simulink model "Example_2_Open"  (Simulink 8.3)
settings: Solver=ode45  StartTime=0.0  StopTime=50  RelTol=1e-3
libraries: simulink x1
settings Model: Creator=NeuControl  LastModifiedBy=Li Jinghao
settings DataIOCC: SignalLoggingSaveFormat=Dataset
settings DebuggingCC: UnderspecifiedInitializationDetection=Simplified  StateNameClashWarn=none
settings GRTTargetCC: CombineOutputUpdateFcns=on  GRTInterface=off

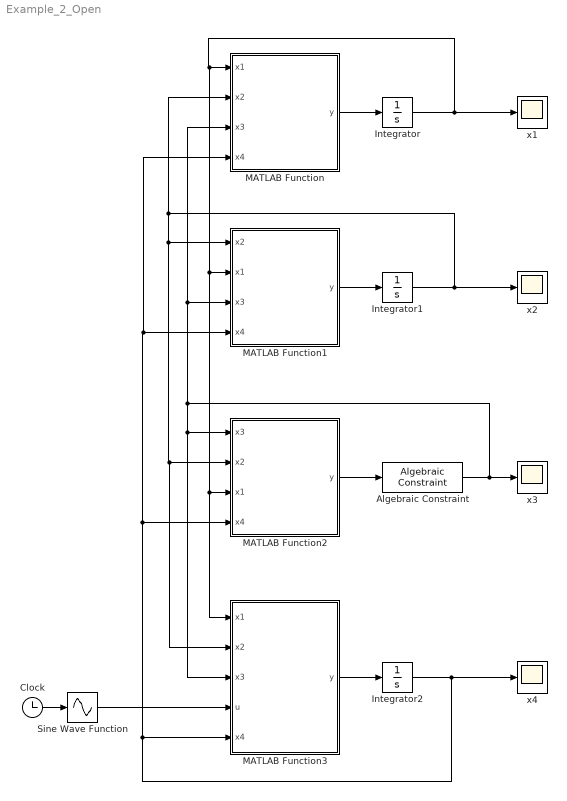
== system Example_2_Open ==
  Algebraic Constraint : simulink/Math Operations/Algebraic Constraint  z0=0
  Clock : Clock
  Integrator : Integrator  InitialCondition=0.5
  Integrator1 : Integrator  InitialCondition=-1
  Integrator2 : Integrator  InitialCondition=2
  MATLAB Function : MATLAB Function  TreatAsAtomicUnit=on
  MATLAB Function1 : MATLAB Function  TreatAsAtomicUnit=on
  MATLAB Function2 : MATLAB Function  TreatAsAtomicUnit=on
  MATLAB Function3 : MATLAB Function  TreatAsAtomicUnit=on
  Sine Wave Function : Sin  TimeSource=Use external signal  Phase=pi/2  SampleTime=0
  x{1..4} (4 alike) : Scope
      x1 settings: SaveName=x1
      x2 settings: SaveName=x2
      x3 settings: SaveName=x3
      x4 settings: SaveName=x4
  wires:
  Integrator/1 -> MATLAB Function3/1(x1), MATLAB Function2/3(x1), MATLAB Function1/2(x1), MATLAB Function/1(x1), x1/1
  MATLAB Function/1(y) -> Integrator/1
  Integrator1/1 -> MATLAB Function/2(x2), MATLAB Function1/1(x2), MATLAB Function3/2(x2), MATLAB Function2/2(x2), x2/1
  MATLAB Function1/1(y) -> Integrator1/1
  Algebraic Constraint/1 -> x3/1, MATLAB Function/3(x3), MATLAB Function1/3(x3), MATLAB Function3/3(x3), MATLAB Function2/1(x3)
  MATLAB Function2/1(y) -> Algebraic Constraint/1
  Integrator2/1 -> x4/1, MATLAB Function3/5(x4), MATLAB Function/4(x4), MATLAB Function1/4(x4), MATLAB Function2/4(x4)
  MATLAB Function3/1(y) -> Integrator2/1
  Clock/1 -> Sine Wave Function/1
  Sine Wave Function/1 -> MATLAB Function3/4(u)

== matlab function MATLAB Function1 ==
  data: x2 input double; x1 input double; y output double; x3 input double; x4 input double
function y = fcn(x2,x1,x3,x4)
%#codegen

gamma=1;
w1=exp(-0.5*(0.5*(x1+5))^2);
w2=exp(-0.5*(0.5*x1)^2);
w3=exp(-0.5*(0.5*(x1-5))^2);
v1=w1/(w1+w2+w3);
v2=w2/(w1+w2+w3);
v3=1-v1-v2;
A1=[-0.5 -0.5 -1 1];
A2=[0.5 -1 0 0.5];
A3=[gamma -1 1 0];
A=v1*A1+v2*A2+v3*A3;
x=[x1;x2;x3;x4];
y = A*x;

== matlab function MATLAB Function ==
  data: x1 input double; y output double; x2 input double; x3 input double; x4 input double
function y = fcn(x1,x2,x3,x4)
%#codegen

beta=-2;
gamma=1;
w1=exp(-0.5*(0.5*(x1+5))^2);
w2=exp(-0.5*(0.5*x1)^2);
w3=exp(-0.5*(0.5*(x1-5))^2);
v1=w1/(w1+w2+w3);
v2=w2/(w1+w2+w3);
v3=1-v1-v2;
A1=[-1 beta 1 -0.5];
A2=[gamma 0.5 0 1];
A3=[-1 beta 0 1];
A=v1*A1+v2*A2+v3*A3;
x=[x1;x2;x3;x4];
y = A*x;

== matlab function MATLAB Function2 ==
  data: x3 input double; x2 input double; x1 input double; y output double; x4 input double
function y = fcn(x3,x2,x1,x4)
%#codegen

w1=exp(-0.5*(0.5*(x1+5))^2);
w2=exp(-0.5*(0.5*x1)^2);
w3=exp(-0.5*(0.5*(x1-5))^2);
v1=w1/(w1+w2+w3);
v2=w2/(w1+w2+w3);
v3=1-v1-v2;
A1=[0 0 -1 1];
A2=[1 0 -1 0.5];
A3=[0 1 -1 1];
A=v1*A1+v2*A2+v3*A3;
x=[x1;x2;x3;x4];
y = A*x;

== matlab function MATLAB Function3 ==
  data: x1 input double; x2 input double; x3 input double; u input double; x4 input double; y output double
function y = fcn(x1,x2,x3,u,x4)
%#codegen


A=[0.5 1 -1.5 1];
x=[x1;x2;x3;x4];
y = A*x+0.5*u;
